simulink model "k1modalitmy"  (Simulink 8.8)
settings: Solver=VariableStepAuto  StartTime=0.0  StopTime=10.0  RelTol=1e-3  EnableMultiTasking=on
libraries: cdsIPCx x34, cdsAdcx0 x1, cdsAdcx1 x1, VISMODAL_MASTER x1, cdsParameters x1
settings Model: SuppressorTable=22 serialization::archive 11 0 3 0 0 0 11 0  Creator=controls  LastModifiedBy=controls
settings DataIOCC: SaveFormat=Dataset  SignalLoggingSaveFormat=Dataset
settings DebuggingCC: UnderspecifiedInitializationDetection=Simplified  MergeDetectMultiDrivingBlocksExec=error  FcnCallInpInsideContextMsg=error  AllowSymbolicDim=off  StateNameClashWarn=none
settings HardwareCC: ProdBitPerPointer=64  ProdBitPerSizeT=64  ProdBitPerPtrDiffT=64  ProdLargestAtomicFloat=Float  ProdIntDivRoundTo=Zero  ProdEndianess=LittleEndian  ProdWordSize=64  ProdHWDeviceType=Intel->x86-64 (Windows64)
settings GRTTargetCC: GeneratePreprocessorConditionals=Use local settings  CombineOutputUpdateFcns=on  GRTInterface=off

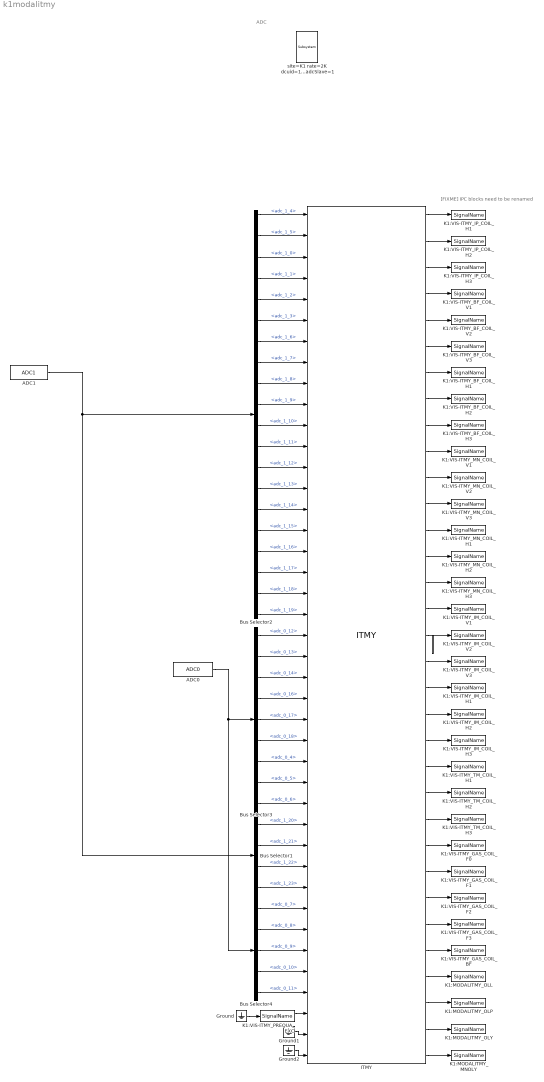
== system k1modalitmy ==
  note: ADC
  note: [FIXME] IPC blocks need to be renamed
  ADC0 : cdsAdcx0/ADC0  Tag=cdsAdc  Description=|
      | type-GSC_16AI64SSA
      | card_num=0
      settings: AttributesFormatString=%<Description>\n%<Tag>
  ADC1 : cdsAdcx1/ADC1  Tag=cdsAdc  Description=|
      | type-GSC_16AI64SSA
      | card_num=1
      settings: AttributesFormatString=%<Description>\n%<Tag>
  Bus Selector1 : BusSelector  OutputSignals=adc_1_20,adc_1_21,adc_1_22,adc_1_23
  Bus Selector2 : BusSelector  OutputSignals=adc_1_4,adc_1_5,adc_1_0,adc_1_1,adc_1_2,adc_1_3,adc_1_6,adc_1_7,adc_1_8,adc_1_9,adc_1_10,adc_1_11,adc_1_12,adc_1_13,adc_1_14,adc_1_15,adc_1_16,adc_1_17,adc_1_18,adc_1_19
  Bus Selector3 : BusSelector  OutputSignals=adc_0_12,adc_0_13,adc_0_14,adc_0_16,adc_0_17,adc_0_18,adc_0_4,adc_0_5,adc_0_6
  Bus Selector4 : BusSelector  OutputSignals=adc_0_7,adc_0_8,adc_0_9,adc_0_10,adc_0_11
  Ground : Ground
  Ground1 : Ground
  Ground2 : Ground
  ITMY : VISMODAL_MASTER/ITMY
  K1:MODALITMY_MNOLY : cdsIPCx/SignalName  Tag=cdsIPCx_SHMEM  Description=Inter-Process Communication via Shared memory.
      settings: AttributesFormatString=%<Tag>
  K1:MODALITMY_OLL : cdsIPCx/SignalName  Tag=cdsIPCx_SHMEM  Description=Inter-Process Communication via Shared memory.
      settings: AttributesFormatString=%<Tag>
  K1:MODALITMY_OLP : cdsIPCx/SignalName  Tag=cdsIPCx_SHMEM  Description=Inter-Process Communication via Shared memory.
      settings: AttributesFormatString=%<Tag>
  K1:MODALITMY_OLY : cdsIPCx/SignalName  Tag=cdsIPCx_SHMEM  Description=Inter-Process Communication via Shared memory.
      settings: AttributesFormatString=%<Tag>
  K1:VIS-ITMY_BF_COIL_H1 : cdsIPCx/SignalName  Tag=cdsIPCx_SHMEM  Description=Inter-Process Communication via Shared memory.
      settings: AttributesFormatString=%<Tag>
  K1:VIS-ITMY_BF_COIL_H2 : cdsIPCx/SignalName  Tag=cdsIPCx_SHMEM  Description=Inter-Process Communication via Shared memory.
      settings: AttributesFormatString=%<Tag>
  K1:VIS-ITMY_BF_COIL_H3 : cdsIPCx/SignalName  Tag=cdsIPCx_SHMEM  Description=Inter-Process Communication via Shared memory.
      settings: AttributesFormatString=%<Tag>
  K1:VIS-ITMY_BF_COIL_V1 : cdsIPCx/SignalName  Tag=cdsIPCx_SHMEM  Description=Inter-Process Communication via Shared memory.
      settings: AttributesFormatString=%<Tag>
  K1:VIS-ITMY_BF_COIL_V2 : cdsIPCx/SignalName  Tag=cdsIPCx_SHMEM  Description=Inter-Process Communication via Shared memory.
      settings: AttributesFormatString=%<Tag>
  K1:VIS-ITMY_BF_COIL_V3 : cdsIPCx/SignalName  Tag=cdsIPCx_SHMEM  Description=Inter-Process Communication via Shared memory.
      settings: AttributesFormatString=%<Tag>
  K1:VIS-ITMY_GAS_COIL_BF : cdsIPCx/SignalName  Tag=cdsIPCx_SHMEM  Description=Inter-Process Communication via Shared memory.
      settings: AttributesFormatString=%<Tag>
  K1:VIS-ITMY_GAS_COIL_F{0..3} (4 alike) : cdsIPCx/SignalName  Tag=cdsIPCx_SHMEM  Description=Inter-Process Communication via Shared memory.
      settings: AttributesFormatString=%<Tag>
  K1:VIS-ITMY_IM_COIL_H1 : cdsIPCx/SignalName  Tag=cdsIPCx_SHMEM  Description=Inter-Process Communication via Shared memory.
      settings: AttributesFormatString=%<Tag>
  K1:VIS-ITMY_IM_COIL_H2 : cdsIPCx/SignalName  Tag=cdsIPCx_SHMEM  Description=Inter-Process Communication via Shared memory.
      settings: AttributesFormatString=%<Tag>
  K1:VIS-ITMY_IM_COIL_H3 : cdsIPCx/SignalName  Tag=cdsIPCx_SHMEM  Description=Inter-Process Communication via Shared memory.
      settings: AttributesFormatString=%<Tag>
  K1:VIS-ITMY_IM_COIL_V1 : cdsIPCx/SignalName  Tag=cdsIPCx_SHMEM  Description=Inter-Process Communication via Shared memory.
      settings: AttributesFormatString=%<Tag>
  K1:VIS-ITMY_IM_COIL_V2 : cdsIPCx/SignalName  Tag=cdsIPCx_SHMEM  Description=Inter-Process Communication via Shared memory.
      settings: AttributesFormatString=%<Tag>
  K1:VIS-ITMY_IM_COIL_V3 : cdsIPCx/SignalName  Tag=cdsIPCx_SHMEM  Description=Inter-Process Communication via Shared memory.
      settings: AttributesFormatString=%<Tag>
  K1:VIS-ITMY_IP_COIL_H1 : cdsIPCx/SignalName  Tag=cdsIPCx_SHMEM  Description=Inter-Process Communication via Shared memory.
      settings: AttributesFormatString=%<Tag>
  K1:VIS-ITMY_IP_COIL_H2 : cdsIPCx/SignalName  Tag=cdsIPCx_SHMEM  Description=Inter-Process Communication via Shared memory.
      settings: AttributesFormatString=%<Tag>
  K1:VIS-ITMY_IP_COIL_H3 : cdsIPCx/SignalName  Tag=cdsIPCx_SHMEM  Description=Inter-Process Communication via Shared memory.
      settings: AttributesFormatString=%<Tag>
  K1:VIS-ITMY_MN_COIL_H1 : cdsIPCx/SignalName  Tag=cdsIPCx_SHMEM  Description=Inter-Process Communication via Shared memory.
      settings: AttributesFormatString=%<Tag>
  K1:VIS-ITMY_MN_COIL_H2 : cdsIPCx/SignalName  Tag=cdsIPCx_SHMEM  Description=Inter-Process Communication via Shared memory.
      settings: AttributesFormatString=%<Tag>
  K1:VIS-ITMY_MN_COIL_H3 : cdsIPCx/SignalName  Tag=cdsIPCx_SHMEM  Description=Inter-Process Communication via Shared memory.
      settings: AttributesFormatString=%<Tag>
  K1:VIS-ITMY_MN_COIL_V1 : cdsIPCx/SignalName  Tag=cdsIPCx_SHMEM  Description=Inter-Process Communication via Shared memory.
      settings: AttributesFormatString=%<Tag>
  K1:VIS-ITMY_MN_COIL_V2 : cdsIPCx/SignalName  Tag=cdsIPCx_SHMEM  Description=Inter-Process Communication via Shared memory.
      settings: AttributesFormatString=%<Tag>
  K1:VIS-ITMY_MN_COIL_V3 : cdsIPCx/SignalName  Tag=cdsIPCx_SHMEM  Description=Inter-Process Communication via Shared memory.
      settings: AttributesFormatString=%<Tag>
  K1:VIS-ITMY_PREQUA_EXC : cdsIPCx/SignalName  Tag=cdsIPCx_SHMEM  Description=Inter-Process Communication via Shared memory.
      settings: AttributesFormatString=%<Tag>
  K1:VIS-ITMY_TM_COIL_H1 : cdsIPCx/SignalName  Tag=cdsIPCx_SHMEM  Description=Inter-Process Communication via Shared memory.
      settings: AttributesFormatString=%<Tag>
  K1:VIS-ITMY_TM_COIL_H2 : cdsIPCx/SignalName  Tag=cdsIPCx_SHMEM  Description=Inter-Process Communication via Shared memory.
      settings: AttributesFormatString=%<Tag>
  K1:VIS-ITMY_TM_COIL_H3 : cdsIPCx/SignalName  Tag=cdsIPCx_SHMEM  Description=Inter-Process Communication via Shared memory.
      settings: AttributesFormatString=%<Tag>
  site=K1 rate=2K dcuid=100 host=k1iy1 specific_cpu=5 adcSlave=1 : cdsParameters/Subsystem  Tag=cdsParameters  Description=|
      | Purpose:                                                                                                                                                                                                                                
      | Provide system parameters to the FE code generator to properly configure the generated EPICS names, rep rate of the FE controller, and the Data Acquisition node ID for proper storage of data from this FE controller.                 
      |                                                                                                                                                                                                                                         
      | Useage:                                                                                                                                                                                                                                 
      | The part NAME field is used to identify the FE parameters. It must be of the form:                                                                                                                                                      
      | site=                                                                                                                                                                                                                                   
      | rate=                                                                                                                                                                                                                                   
      | dcuid=                                                                                                                                                                                                                                  
      |                                                                                                                                                                                                                                         
      | Where:                                                                                                                                                                                                                                  
      | site= argument may be H1, H2, L1, M1, G1, either as a single argument or multiple, for example site=H1,H2. These are the only names allowed. These will become the first two characters of all EPICS and signal names (for example G1:).
      |                                                                                                                                                                                                                                         
      | rate= may be 2K, 16K, 32K, or 64K                                                                                                                                                                                                       
      |                                                                                                                                                                                                                                         
      | dcuid= is site specific ie it must be unique at each site.
      settings: AttributesFormatString=%<Tag>
  wires:
  ITMY/10 -> K1:VIS-ITMY_MN_COIL_V1/1
  ITMY/11 -> K1:VIS-ITMY_MN_COIL_V2/1
  ITMY/12 -> K1:VIS-ITMY_MN_COIL_V3/1
  ITMY/13 -> K1:VIS-ITMY_MN_COIL_H1/1
  ITMY/14 -> K1:VIS-ITMY_MN_COIL_H2/1
  ITMY/15 -> K1:VIS-ITMY_MN_COIL_H3/1
  ITMY/16 -> K1:VIS-ITMY_IM_COIL_V1/1
  ITMY/17 -> K1:VIS-ITMY_IM_COIL_V2/1
  ITMY/18 -> K1:VIS-ITMY_IM_COIL_V3/1
  ITMY/19 -> K1:VIS-ITMY_IM_COIL_H1/1
  ITMY/20 -> K1:VIS-ITMY_IM_COIL_H2/1
  ITMY/21 -> K1:VIS-ITMY_IM_COIL_H3/1
  ITMY/22 -> K1:VIS-ITMY_TM_COIL_H1/1
  ITMY/23 -> K1:VIS-ITMY_TM_COIL_H2/1
  ITMY/24 -> K1:VIS-ITMY_TM_COIL_H3/1
  ITMY/1 -> K1:VIS-ITMY_IP_COIL_H1/1
  ITMY/2 -> K1:VIS-ITMY_IP_COIL_H2/1
  ITMY/3 -> K1:VIS-ITMY_IP_COIL_H3/1
  ITMY/4 -> K1:VIS-ITMY_BF_COIL_V1/1
  ITMY/5 -> K1:VIS-ITMY_BF_COIL_V2/1
  ITMY/6 -> K1:VIS-ITMY_BF_COIL_V3/1
  ITMY/7 -> K1:VIS-ITMY_BF_COIL_H1/1
  ITMY/8 -> K1:VIS-ITMY_BF_COIL_H2/1
  ITMY/9 -> K1:VIS-ITMY_BF_COIL_H3/1
  ADC1/1 -> Bus Selector1/1, Bus Selector2/1
  Bus Selector2/1 -> ITMY/1  "<adc_1_4>"
  Bus Selector2/2 -> ITMY/2  "<adc_1_5>"
  Bus Selector2/3 -> ITMY/3  "<adc_1_0>"
  Bus Selector2/4 -> ITMY/4  "<adc_1_1>"
  Bus Selector2/5 -> ITMY/5  "<adc_1_2>"
  Bus Selector2/6 -> ITMY/6  "<adc_1_3>"
  Bus Selector2/7 -> ITMY/7  "<adc_1_6>"
  Bus Selector2/8 -> ITMY/8  "<adc_1_7>"
  Bus Selector2/9 -> ITMY/9  "<adc_1_8>"
  Bus Selector2/10 -> ITMY/10  "<adc_1_9>"
  Bus Selector2/11 -> ITMY/11  "<adc_1_10>"
  Bus Selector2/12 -> ITMY/12  "<adc_1_11>"
  Bus Selector2/13 -> ITMY/13  "<adc_1_12>"
  Bus Selector2/14 -> ITMY/14  "<adc_1_13>"
  Bus Selector2/15 -> ITMY/15  "<adc_1_14>"
  Bus Selector2/16 -> ITMY/16  "<adc_1_15>"
  Bus Selector2/17 -> ITMY/17  "<adc_1_16>"
  Bus Selector2/18 -> ITMY/18  "<adc_1_17>"
  Bus Selector2/19 -> ITMY/19  "<adc_1_18>"
  Bus Selector2/20 -> ITMY/20  "<adc_1_19>"
  ADC0/1 -> Bus Selector4/1, Bus Selector3/1
  Bus Selector3/1 -> ITMY/21  "<adc_0_12>"
  Bus Selector3/2 -> ITMY/22  "<adc_0_13>"
  Bus Selector3/3 -> ITMY/23  "<adc_0_14>"
  Bus Selector3/4 -> ITMY/24  "<adc_0_16>"
  Bus Selector3/5 -> ITMY/25  "<adc_0_17>"
  Bus Selector3/6 -> ITMY/26  "<adc_0_18>"
  Bus Selector3/7 -> ITMY/27  "<adc_0_4>"
  Bus Selector3/8 -> ITMY/28  "<adc_0_5>"
  Bus Selector3/9 -> ITMY/29  "<adc_0_6>"
  Bus Selector1/1 -> ITMY/30  "<adc_1_20>"
  Bus Selector1/2 -> ITMY/31  "<adc_1_21>"
  Bus Selector1/3 -> ITMY/32  "<adc_1_22>"
  Bus Selector1/4 -> ITMY/33  "<adc_1_23>"
  ITMY/25 -> K1:VIS-ITMY_GAS_COIL_F0/1
  ITMY/26 -> K1:VIS-ITMY_GAS_COIL_F1/1
  ITMY/27 -> K1:VIS-ITMY_GAS_COIL_F2/1
  ITMY/28 -> K1:VIS-ITMY_GAS_COIL_F3/1
  ITMY/29 -> K1:VIS-ITMY_GAS_COIL_BF/1
  Bus Selector4/1 -> ITMY/34  "<adc_0_7>"
  Bus Selector4/2 -> ITMY/35  "<adc_0_8>"
  Bus Selector4/3 -> ITMY/36  "<adc_0_9>"
  Bus Selector4/4 -> ITMY/37  "<adc_0_10>"
  Bus Selector4/5 -> ITMY/38  "<adc_0_11>"
  K1:VIS-ITMY_PREQUA_EXC/1 -> ITMY/39
  Ground/1 -> K1:VIS-ITMY_PREQUA_EXC/1
  Ground1/1 -> ITMY/40
  Ground2/1 -> ITMY/41
  ITMY/31 -> K1:MODALITMY_OLP/1
  ITMY/32 -> K1:MODALITMY_OLY/1
  ITMY/30 -> K1:MODALITMY_OLL/1
  ITMY/33 -> K1:MODALITMY_MNOLY/1
